simulink model "PLL_lineal_a"  (R2024a)
settings: Solver=VariableStepAuto  StartTime=0.0  StopTime=10  FixedStep=0.1  RelTol=1e-5  EnableMultiTasking=on
model workspace (MAT data in the model file):
  Cf = 1e-06
  Cvco = 5e-09
  Kvco = 320
  Kvco_l = 2010.6192983
  N = 32
  R1 = 10000
  R2 = 200000
  Rvco = 100000
  Ts = 5e-05
  VDD = 10
  fi = 50
  wi = 314.159265359
libraries: simulink x1
settings Model: ModifiedByFormat=The MathWorks, Inc.  Creator=The MathWorks, Inc.  LastModifiedBy=The MathWorks, Inc.
settings SolverCC: MaxConsecutiveZCs=100000  ZeroCrossAlgorithm=Adaptive  AlgebraicLoopSolver=TrustRegion
settings DataIOCC: LimitDataPoints=on  MaxDataPoints=100000  SaveFormat=Array  ReturnWorkspaceOutputs=off
settings OptimizationCC: ReuseModelBlockBuffer=off  ExpressionDepthLimit=2147483647  LifeSpan=inf
settings DebuggingCC: FcnCallInpInsideContextMsg=warning  UnconnectedInputMsg=warning  UnconnectedOutputMsg=warning  UnconnectedLineMsg=warning  StateNameClashWarn=warning  SFUnexpectedBacktrackingDiag=warning  SFNoUnconditionalDefaultTransitionDiag=warning  SFExecutionAtInitializationDiag=none  ArithmeticOperatorsInVariantConditions=warning
settings HardwareCC: ProdBitPerPointer=32  ProdBitPerSizeT=32  ProdBitPerPtrDiffT=32  ProdLargestAtomicFloat=None  ProdIntDivRoundTo=Undefined  ProdEndianess=Unspecified  ProdWordSize=32  ProdHWDeviceType=32-bit Generic
settings ModelReferenceCC: EnableRefExpFcnMdlSchedulingChecks=on  PropagateSignalLabelsOutOfModel=off
settings SFSimCC: SimUseLocalCustomCode=off  CustomCodeUndefinedFunction=UseInterfaceOnly
settings RTWCC: RTWUseLocalCustomCode=off  GPUComputeCapability=3.5  DLArmComputeVersion=19.05
settings CodeAppCC: StateflowObjectComments=on
settings GRTTargetCC: TargetLangStandard=C89/C90 (ANSI)  CombineOutputUpdateFcns=off  GRTInterface=on
settings ConfigComp: CovMetricSettings=dw  CovSaveCumulativeToWorkspaceVar=on  CovSaveSingleToWorkspaceVar=on  CovExternalEMLEnable=off

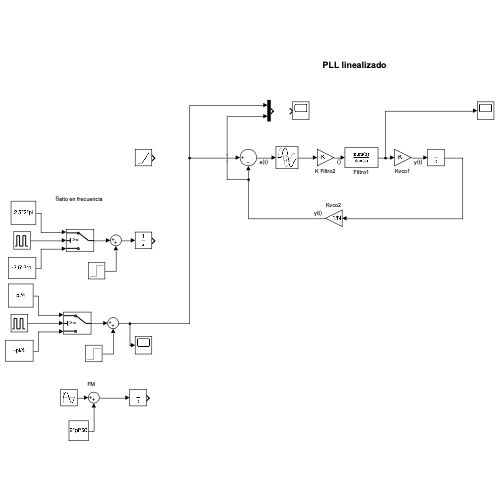
[thumbnail: Simulink's stored preview of the top-level diagram]
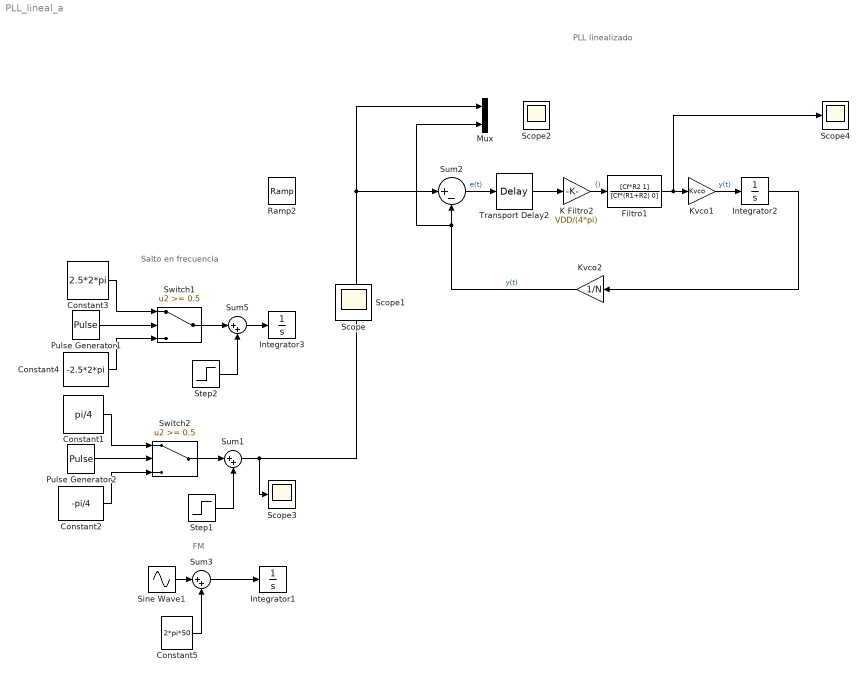
== system PLL_lineal_a ==
  note: PLL linealizado
  note: Salto en frecuencia
  note: FM
  Constant1 : Constant  Value=pi/4
  Constant2 : Constant  Value=-pi/4
  Constant3 : Constant  Value=2.5*2*pi
  Constant4 : Constant  Value=-2.5*2*pi
  Constant5 : Constant  Value=2*pi*50
  Filtro1 : TransferFcn  Numerator=[Cf*R2 1]  Denominator=[Cf*(R1+R2) 0]
  Integrator1 : Integrator
  Integrator2 : Integrator
  Integrator3 : Integrator
  K Filtro2 : Gain  Gain=VDD/(4*pi)
  Kvco1 : Gain  Gain=Kvco
  Kvco2 : Gain  Gain=1/N
  Mux : Mux  Inputs=2
  Pulse Generator1 : DiscretePulseGenerator  PulseType=Time based  Period=1  PulseWidth=50
  Pulse Generator2 : DiscretePulseGenerator  PulseType=Time based  PulseWidth=50
  Ramp2 : simulink/Sources/Ramp  slope=2*pi*50  start=0  InitialOutput=0
  Scope{,1..4} (5 alike) : Scope
  Sine Wave1 : Sin  Amplitude=5*2*pi  Frequency=2*pi*4  SampleTime=0
  Step1 : Step  Time=0  After=pi/2  SampleTime=0
  Step2 : Step  Time=0  After=2*pi*50  SampleTime=0
  Sum1 : Sum  Inputs=|++
  Sum2 : Sum  Inputs=|+-
  Sum3 : Sum  Inputs=|++
  Sum5 : Sum  Inputs=|++
  Switch1 : Switch  Threshold=0.5  SaturateOnIntegerOverflow=off  InputSameDT=off
  Switch2 : Switch  Threshold=0.5  SaturateOnIntegerOverflow=off  InputSameDT=off
  Transport Delay2 : TransportDelay  DelayTime=1/(2*fi)
  wires:
  Integrator2/1 -> Kvco2/1
  Kvco1/1 -> Integrator2/1  "y(t)"
  K Filtro2/1 -> Filtro1/1  "()"
  Filtro1/1 -> Scope4/1, Kvco1/1
  Kvco2/1 -> Mux/2, Sum2/2  "y(t)"
  Sum2/1 -> Transport Delay2/1  "e(t)"
  Transport Delay2/1 -> K Filtro2/1
  Switch1/1 -> Sum5/1
  Constant3/1 -> Switch1/1
  Constant4/1 -> Switch1/3
  Step2/1 -> Sum5/2
  Sum5/1 -> Integrator3/1
  Pulse Generator1/1 -> Switch1/2
  Constant1/1 -> Switch2/1
  Constant2/1 -> Switch2/3
  Pulse Generator2/1 -> Switch2/2
  Switch2/1 -> Sum1/1
  Step1/1 -> Sum1/2
  Sine Wave1/1 -> Sum3/1
  Constant5/1 -> Sum3/2
  Sum3/1 -> Integrator1/1
  Sum1/1 -> Scope3/1, Mux/1, Sum2/1
